simulink model "QPSK_OFDM_Rayleigh"  (R2019b)
settings: Solver=VariableStepAuto  StartTime=0.0  StopTime=5  RelTol=1e-3
undefined symbols (not defined in the file or in its folder): doppler
libraries: commchan3 x2, commutil2 x2, dspxfrm3 x2, commdigbbndpm3 x2, commrandsrc3 x1, commsink2 x1
settings Model: Creator=Nikhil  LastModifiedBy=Nikhil

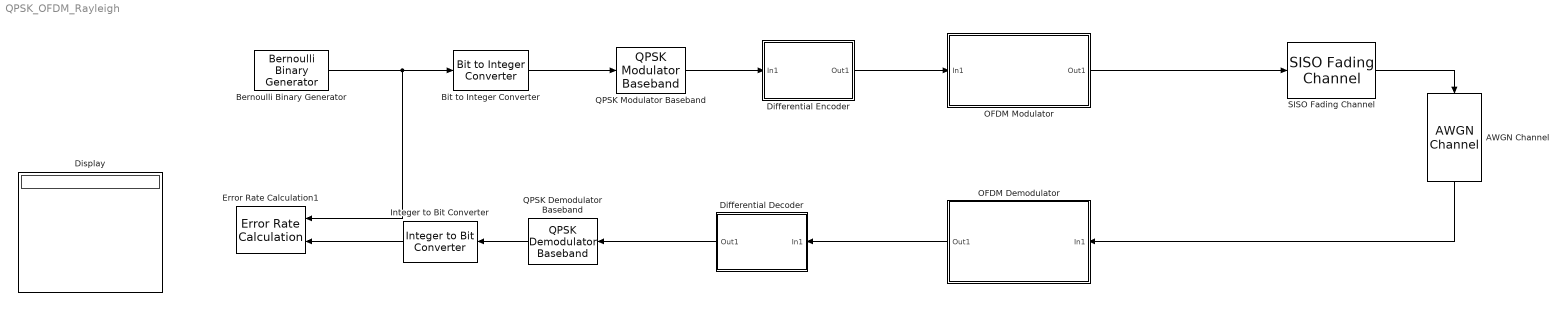
== system QPSK_OFDM_Rayleigh ==
  AWGN Channel : commchan3/AWGN Channel  InputProcessing=Columns as channels (frame based)  seed=117  noiseMode="Signal to noise ratio  (SNR)"  EbNodB=10  EsNodB=10  SNRdB=s  bitsPerSym=1  Ps=1  Tsym=1  variance=1
      settings: SourceProductName=Communications Toolbox
  Bernoulli Binary Generator : commrandsrc3/Bernoulli Binary Generator  ProbabilityOfZero=0.5  SeedSource=Auto  Seed=322  SampleTime=5e-7  SamplesPerFrame=104  OutputDataType=uint8  SimulateUsing=Interpreted execution
      settings: SourceProductName=Communications Toolbox
  Bit to Integer Converter : commutil2/Bit to Integer Converter  nbits=2  bitOrder=MSB first  signedOutputValues=Unsigned  outDtype=Inherit via internal rule  outDtypeSigned=Inherit via internal rule
      settings: SourceProductName=Communications Toolbox
  Differential Decoder : Subsystem
  Differential Encoder : Subsystem
  Display : Display
  Error Rate Calculation1 : commsink2/Error Rate Calculation  N=0  st_delay=0  cp_mode=Entire frame  subframe=[]  PMode=Workspace  WsName=ErrorVec  RsMode2=off  stop=off  numErr=100  maxBits=1e6
      settings: SourceProductName=Communications Toolbox
  Integer to Bit Converter : commutil2/Integer to Bit Converter  nbits=2  signedInputValues=Unsigned  bitOrder=MSB first  outDtype=Inherit via internal rule
      settings: SourceProductName=Communications Toolbox
  OFDM Demodulator : Subsystem
  OFDM Modulator : Subsystem
  QPSK Demodulator Baseband : commdigbbndpm3/QPSK Demodulator Baseband  OutType=Integer  DecType=Hard decision  VarSource=Dialog  Variance=1  Dec=Gray  Ph=pi/4  outDtype1=Inherit via internal rule  outDtype2=Inherit via internal rule  derotateFactorWordLen=16  derotateFactorDataTypeStr=Inherit: Same word length as input  derotateFactorLastDataTypeStr=Inherit: Same word length as input
      settings: SourceProductName=Communications Toolbox
  QPSK Modulator Baseband : commdigbbndpm3/QPSK Modulator Baseband  InType=Integer  Enc=Gray  Ph=pi/4  outDtype=Inherit via back propagation  outWordLen=16  outUDDataType=sfix(16)  outFracLenMode=Best precision  outFracLen=15  outDataTypeStr=Inherit: Inherit via back propagation  outLastDataTypeStr=Inherit: Inherit via back propagation
      settings: SourceProductName=Communications Toolbox
  SISO Fading Channel : commchan3/SISO Fading Channel  InheritSampleRate=on  SampleRate=1  PathDelays=[0 1.8e-5 1.3e-5 1.1e-5 1e-5 1.4e-5]  AveragePathGains=[0,0,0,0,0,0]  NormalizePathGains=on  FadingDistribution=Rayleigh  KFactor=3  DirectPathDopplerShift=0  DirectPathInitialPhase=0  MaximumDopplerShift=100  DopplerSpectrum=doppler('Flat')  RandomStream=mt19937ar with seed  Seed=77  PathGainsOutputPort=off  ChannelFilterDelayOutputPort=off  SimulateUsing=Interpreted execution  Visualization=Off  PathsForDopplerDisplay=1  SamplesToDisplay=25%
      settings: SourceProductName=Communications Toolbox
  wires:
  Bit to Integer Converter/1 -> QPSK Modulator Baseband/1
  Integer to Bit Converter/1 -> Error Rate Calculation1/2
  QPSK Demodulator Baseband/1 -> Integer to Bit Converter/1
  Differential Decoder/1(Out1) -> QPSK Demodulator Baseband/1
  Bernoulli Binary Generator/1 -> Error Rate Calculation1/1, Bit to Integer Converter/1
  QPSK Modulator Baseband/1 -> Differential Encoder/1(In1)
  SISO Fading Channel/1 -> AWGN Channel/1
  Differential Encoder/1(Out1) -> OFDM Modulator/1(In1)
  OFDM Modulator/1(Out1) -> SISO Fading Channel/1
  OFDM Demodulator/1(Out1) -> Differential Decoder/1(In1)
  AWGN Channel/1 -> OFDM Demodulator/1(In1)

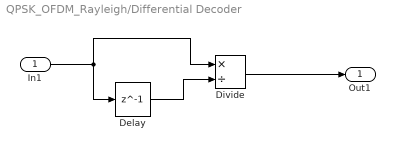
== system QPSK_OFDM_Rayleigh/Differential Decoder ==
  In1 : Inport
  Delay : Delay  DelayLength=1  InitialCondition=1
  Divide : Product  Inputs=*/
  Out1 : Outport
  wires:
  In1/1 -> Delay/1, Divide/1
  Divide/1 -> Out1/1
  Delay/1 -> Divide/2

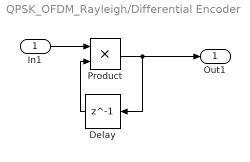
== system QPSK_OFDM_Rayleigh/Differential Encoder ==
  In1 : Inport
  Delay : Delay  DelayLength=1  InitialCondition=1
  Product : Product
  Out1 : Outport
  wires:
  In1/1 -> Product/1
  Product/1 -> Delay/1, Out1/1
  Delay/1 -> Product/2

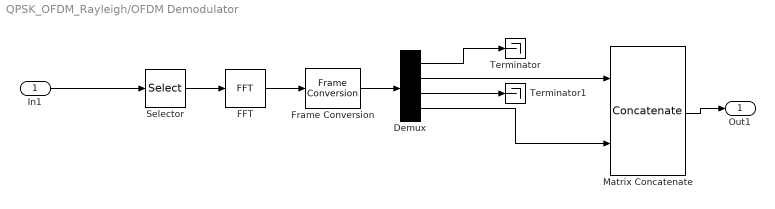
== system QPSK_OFDM_Rayleigh/OFDM Demodulator ==
  In1 : Inport
  Demux : Demux  Outputs=[1 26 11 26]
  FFT : dspxfrm3/FFT  FFTImplementation=Auto  CompMethod=Table lookup  TableOpt=NEW  TableOptActive=Speed  BitRevOrder=off  Normalize=off  InheritFFTLength=on  FFTLength=104  WrapInput=off  roundingMode=Floor  overflowMode=off  firstCoeffDataTypeStr=Inherit: Same word length as input  firstCoeffLastDataTypeStr=Inherit: Same word length as input  outputMin=[]  outputMax=[]
  Frame Conversion : FrameConversion  OutFrame=Sample-based
  Matrix Concatenate : Concatenate  ConcatenateDimension=2
  Selector : Selector  InputPortWidth=80  IndexOptions=Index vector (dialog)  Indices=[17:80]  OutputSizes=1
  Terminator : Terminator
  Terminator1 : Terminator
  Out1 : Outport
  wires:
  In1/1 -> Selector/1
  Selector/1 -> FFT/1
  FFT/1 -> Frame Conversion/1
  Frame Conversion/1 -> Demux/1
  Demux/3 -> Terminator1/1
  Demux/1 -> Terminator/1
  Matrix Concatenate/1 -> Out1/1
  Demux/2 -> Matrix Concatenate/1
  Demux/4 -> Matrix Concatenate/2

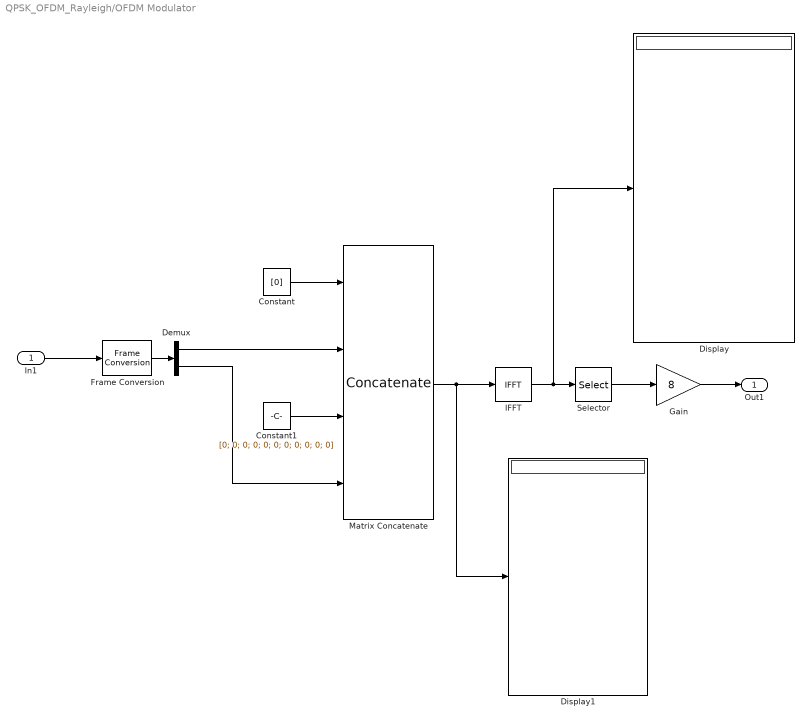
== system QPSK_OFDM_Rayleigh/OFDM Modulator ==
  In1 : Inport
  Constant : Constant  Value=[0]
  Constant1 : Constant  Value=[0; 0; 0; 0; 0; 0; 0; 0; 0; 0; 0]
  Demux : Demux  Outputs=2
  Display : Display
  Display1 : Display
  Frame Conversion : FrameConversion  OutFrame=Sample-based
  Gain : Gain  Gain=8
  IFFT : dspxfrm3/IFFT  FFTImplementation=Auto  CompMethod=Table lookup  TableOpt=NEW  TableOptActive=Speed  BitRevOrder=off  cs_in=off  Normalize=on  InheritFFTLength=on  FFTLength=80  WrapInput=off  mode=Complex  outSamplingMode=Sample based  roundingMode=Floor  overflowMode=off  firstCoeffDataTypeStr=Inherit: Same word length as input  firstCoeffLastDataTypeStr=Inherit: Same word length as input  outputMin=[]  outputMax=[]
      settings: SourceProductName=DSP System Toolbox
  Matrix Concatenate : Concatenate  NumInputs=4  ConcatenateDimension=2
  Selector : Selector  InputPortWidth=64  IndexOptions=Index vector (dialog)  Indices=[49:64 1:64]  OutputSizes=16
  Out1 : Outport
  wires:
  In1/1 -> Frame Conversion/1
  Frame Conversion/1 -> Demux/1
  Demux/1 -> Matrix Concatenate/2
  Demux/2 -> Matrix Concatenate/4
  Constant/1 -> Matrix Concatenate/1
  Constant1/1 -> Matrix Concatenate/3
  Matrix Concatenate/1 -> Display1/1, IFFT/1
  IFFT/1 -> Display/1, Selector/1
  Gain/1 -> Out1/1
  Selector/1 -> Gain/1
